simulink model "quadplane_control_dev"  (R2023a)
settings: Solver=FixedStepAuto  StartTime=0.0  StopTime=10.0  FixedStep=0.01  RelTol=1e-3
undefined symbols (not defined in the file or in its folder): Aircraft, DiscIntNeverNeededParam, framePeriod_s, frameRate_hz, InitCond
libraries: simulink x8, eeGeneralControl x6, slpidlib x3, fuzblock x1
(part 2 of 3)

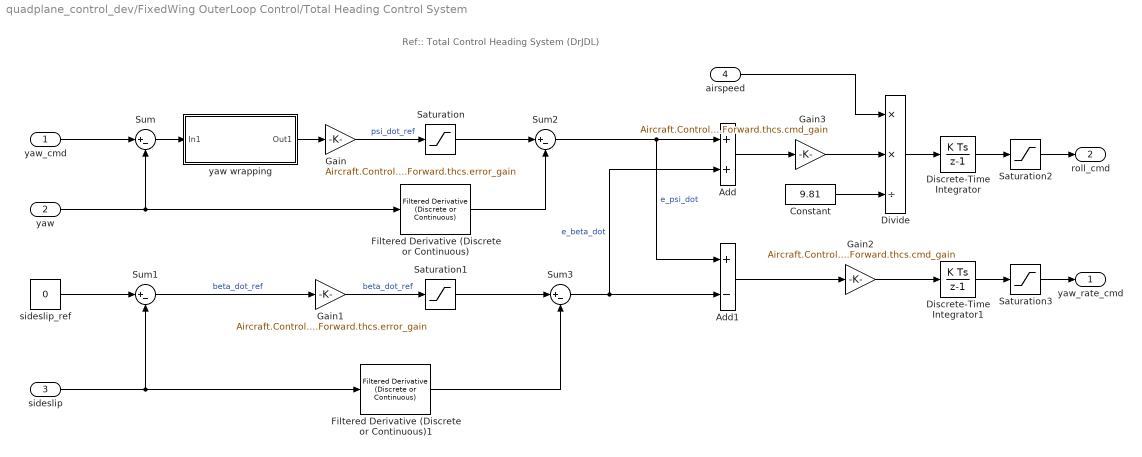
== system quadplane_control_dev/FixedWing OuterLoop Control/Total Heading Control System ==
  note: Ref:: Total Control Heading System (DrJDL)
  yaw_cmd : Inport
  yaw : Inport  Port=2
  sideslip : Inport  Port=3
  airspeed : Inport  Port=4
  " yaw wrapping" : Subsystem
  Add : Sum
  Add1 : Sum  Inputs=+-
  Constant : Constant  Value=9.81  OutDataTypeStr=single
  Discrete-Time Integrator : DiscreteIntegrator  SampleTime=-1  ICPrevOutput=DiscIntNeverNeededParam  ICPrevScaledInput=DiscIntNeverNeededParam
  Discrete-Time Integrator1 : DiscreteIntegrator  SampleTime=-1  ICPrevOutput=DiscIntNeverNeededParam  ICPrevScaledInput=DiscIntNeverNeededParam
  Divide : Product  Inputs=**/
  Filtered Derivative (Discrete or Continuous) : eeGeneralControl/Filtered Derivative (Discrete or Continuous)  K=1  T=0.1  B=inf  A=-inf  minRatio=10  init_option=Inherited from block input  x0=0  Ts=-1
      settings: LibrarySourceBlock=|
      | ee_sl_lib/General Control/Filtered Derivative
      | (Discrete or Continuous)
  Filtered Derivative (Discrete or Continuous)1 : eeGeneralControl/Filtered Derivative (Discrete or Continuous)  K=1  T=0.05  B=inf  A=-inf  minRatio=10  init_option=Inherited from block input  x0=0  Ts=-1
      settings: LibrarySourceBlock=|
      | ee_sl_lib/General Control/Filtered Derivative
      | (Discrete or Continuous)
  Gain : Gain  Gain=Aircraft.Control.Forward.thcs.error_gain
  Gain1 : Gain  Gain=Aircraft.Control.Forward.thcs.error_gain
  Gain2 : Gain  Gain=Aircraft.Control.Forward.thcs.cmd_gain
  Gain3 : Gain  Gain=Aircraft.Control.Forward.thcs.cmd_gain
  Saturation : Saturate  UpperLimit=Aircraft.Control.Forward.thcs.psi_dot_ref  LowerLimit=-Aircraft.Control.Forward.thcs.psi_dot_ref  OutDataTypeStr=single
  Saturation1 : Saturate  UpperLimit=Aircraft.Control.Forward.thcs.beta_dot_ref_limit  LowerLimit=-Aircraft.Control.Forward.thcs.beta_dot_ref_limit  OutDataTypeStr=single
  Saturation2 : Saturate  UpperLimit=Aircraft.Control.Forward.max_roll_rad  LowerLimit=-Aircraft.Control.Forward.max_roll_rad  OutDataTypeStr=single
  Saturation3 : Saturate  UpperLimit=Aircraft.Control.Forward.max_yaw_rate  LowerLimit=-Aircraft.Control.Forward.max_yaw_rate  OutDataTypeStr=single
  Sum{,1..3} (4 alike) : Sum  Inputs=|+-
  sideslip_ref : Constant  Value=0  OutDataTypeStr=single
  yaw_rate_cmd : Outport
  roll_cmd : Outport  Port=2
  wires:
  yaw_cmd/1 -> Sum/1
  yaw/1 -> Filtered Derivative (Discrete or Continuous)/1, Sum/2
  Sum/1 -> " yaw wrapping"/1(In1)
  sideslip_ref/1 -> Sum1/1
  sideslip/1 -> Filtered Derivative (Discrete or Continuous)1/1, Sum1/2
  Gain/1 -> Saturation/1  "psi_dot_ref"
  Gain1/1 -> Saturation1/1  "beta_dot_ref"
  Saturation/1 -> Sum2/1
  Filtered Derivative (Discrete or Continuous)/1 -> Sum2/2
  Sum2/1 -> Add1/1, Add/1  "e_psi_dot"
  Saturation1/1 -> Sum3/1
  Filtered Derivative (Discrete or Continuous)1/1 -> Sum3/2
  Sum3/1 -> Add/2, Add1/2  "e_beta_dot"
  Add1/1 -> Gain2/1
  Gain2/1 -> Discrete-Time Integrator1/1
  Discrete-Time Integrator1/1 -> Saturation3/1
  Add/1 -> Gain3/1
  Gain3/1 -> Divide/2
  Constant/1 -> Divide/3
  Divide/1 -> Discrete-Time Integrator/1
  airspeed/1 -> Divide/1
  Discrete-Time Integrator/1 -> Saturation2/1
  " yaw wrapping"/1(Out1) -> Gain/1
  Saturation2/1 -> roll_cmd/1
  Saturation3/1 -> yaw_rate_cmd/1
  Sum1/1 -> Gain1/1  "beta_dot_ref"

== system quadplane_control_dev/Hover Inner Loop/Attitude Control ==
  note: Limiting the pqr_ref to 2/-2 radps
  yaw_rate_ref : Inport
  roll_pitch_ref : Inport  Port=2
  roll_pitch_yaw : Inport  Port=3
  Gain1 : Gain  Gain=Aircraft.Control.Hover_v2.att_gain
  Mux : Mux  Inputs=2
  Saturation : Saturate  UpperLimit=Aircraft.Control.Hover.pqr_limit  LowerLimit=-Aircraft.Control.Hover.pqr_limit
  Selector : Selector  InputPortWidth=3  IndexOptions=Index vector (dialog)  Indices=[1 2]  OutputSizes=1
  Sum : Sum  Inputs=|+-  AccumDataTypeStr=single
  pqr_ref1 : Outport
  wires:
  roll_pitch_ref/1 -> Sum/1
  Sum/1 -> Gain1/1  "roll_pitch_err"
  Mux/1 -> Saturation/1
  Saturation/1 -> pqr_ref1/1
  Selector/1 -> Sum/2
  roll_pitch_yaw/1 -> Selector/1
  Gain1/1 -> Mux/1
  yaw_rate_ref/1 -> Mux/2

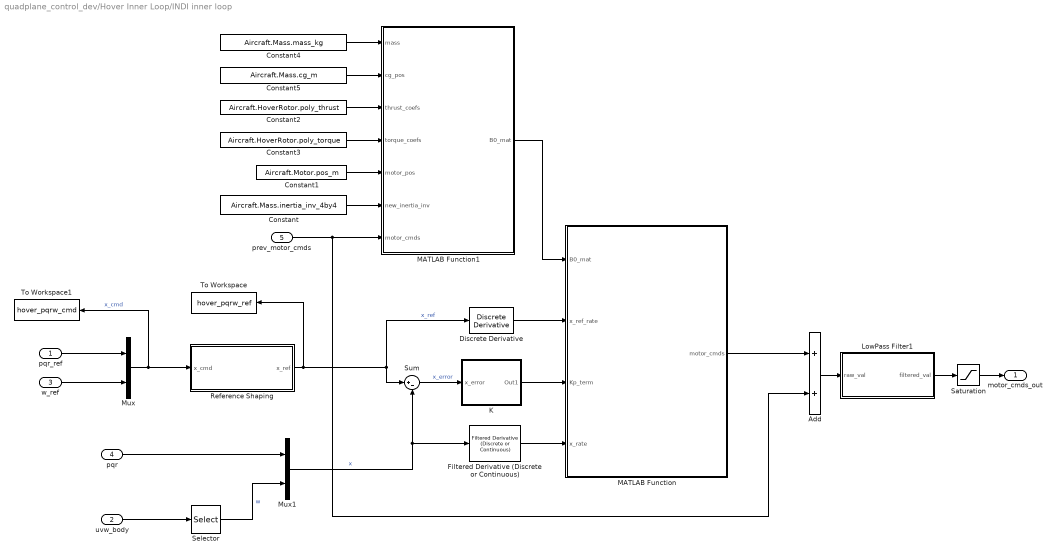
== system quadplane_control_dev/Hover Inner Loop/INDI inner loop ==
  pqr_ref : Inport
  uvw_body : Inport  Port=2
  w_ref : Inport  Port=3
  pqr : Inport  Port=4
  prev_motor_cmds : Inport  Port=5
  Add : Sum
  Constant : Constant  Value=Aircraft.Mass.inertia_inv_4by4  OutDataTypeStr=single
  Constant1 : Constant  Value=Aircraft.Motor.pos_m  OutDataTypeStr=single
  Constant2 : Constant  Value=Aircraft.HoverRotor.poly_thrust  OutDataTypeStr=single
  Constant3 : Constant  Value=Aircraft.HoverRotor.poly_torque  OutDataTypeStr=single
  Constant4 : Constant  Value=Aircraft.Mass.mass_kg
  Constant5 : Constant  Value=Aircraft.Mass.cg_m
  Discrete Derivative : simulink/Discrete/Discrete Derivative  gainval=1.0  ICPrevScaledInput=0.0  OutMin=[]  OutMax=[]  OutDataType=fixdt(1, 16)  OutScaling=2^-10  DoSatur=off
  Filtered Derivative (Discrete or Continuous) : eeGeneralControl/Filtered Derivative (Discrete or Continuous)  K=1  T=0.01  B=inf  A=-inf  minRatio=10  init_option=Inherited from block input  x0=0  Ts=-1
      settings: LibrarySourceBlock=|
      | ee_sl_lib/General Control/Filtered Derivative
      | (Discrete or Continuous)
  K : Subsystem
  LowPass Filter1 : Subsystem
      settings: PortSchema="{\"entries\":[{\"content\":{\"sides\":[{\"content\":{\"connectorIds\":[\"Out1\"]},\"type\":\"ConnectorPlacement.EquallySpacedRectSide\",\"uuid\":\"91cc3e13-2b14-472d-8884-d1975898cd34\"},{\"content\":{\"connectorIds\":[\"In1\"],\"side\":\"RIGHT\"},\"type\":\"ConnectorPlacement.EquallySpacedRectSide\",\"uuid\":\"ce6b3021-6e32-4737-8c8e-25014706d3dd\"},{\"content\":{\"side\":\"TOP\"},\"type\":\"ConnectorPlacement.EquallySpacedRectSide\",\"uuid\":\"ad734f0b-b067-43e6-a641-0e0955250a7f\"},{\"content\":{\"side\":\"BOTTOM\"},\"type\":\"ConnectorPlacement.EquallySpacedRectSide\",\"uuid\":\"618c62c8-d4e2-4678-9fe1-905e2f147d5d\"}]},\"type\":\"ConnectorPlacement.EquallySpacedConnector\",\"uuid\":\"c0097053-d36a-473a-84fb-0616f69f4bc5\"}],\"packageUris\":[\"http://schema.mathworks.com/mf0/Connector/R2020b\"],\"version\":\"1.0\"}"
  MATLAB Function : MATLAB Function  TreatAsAtomicUnit=on
  MATLAB Function1 : MATLAB Function  TreatAsAtomicUnit=on
  Mux : Mux  Inputs=2
  Mux1 : Mux  Inputs=2
  Reference Shaping : Subsystem
  Saturation : Saturate  UpperLimit=1  LowerLimit=0.2
  Selector : Selector  InputPortWidth=3  IndexOptions=Index vector (dialog)  Indices=3  OutputSizes=1
  Sum : Sum  Inputs=|+-  OutDataTypeStr=single
  To Workspace : ToWorkspace  VariableName=hover_pqrw_ref  SaveFormat=Timeseries  SampleTime=-1
  To Workspace1 : ToWorkspace  VariableName=hover_pqrw_cmd  SaveFormat=Timeseries  SampleTime=-1
  motor_cmds_out : Outport
  wires:
  Constant2/1 -> MATLAB Function1/3(thrust_coefs)
  MATLAB Function/1(motor_cmds) -> Add/1
  uvw_body/1 -> Selector/1
  Discrete Derivative/1 -> MATLAB Function/2(x_ref_rate)
  Constant4/1 -> MATLAB Function1/1(mass)
  Constant3/1 -> MATLAB Function1/4(torque_coefs)
  pqr_ref/1 -> Mux/1
  pqr/1 -> Mux1/1
  Constant1/1 -> MATLAB Function1/5(motor_pos)
  Mux1/1 -> Filtered Derivative (Discrete or Continuous)/1, Sum/2  "x"
  Constant/1 -> MATLAB Function1/6(new_inertia_inv)
  MATLAB Function1/1(B0_mat) -> MATLAB Function/1(B0_mat)
  Constant5/1 -> MATLAB Function1/2(cg_pos)
  Selector/1 -> Mux1/2  "w"
  w_ref/1 -> Mux/2
  Reference Shaping/1(x_ref) -> To Workspace/1, Discrete Derivative/1, Sum/1  "x_ref"
  Filtered Derivative (Discrete or Continuous)/1 -> MATLAB Function/4(x_rate)
  Mux/1 -> To Workspace1/1, Reference Shaping/1(x_cmd)  "x_cmd"
  Saturation/1 -> motor_cmds_out/1
  Add/1 -> LowPass Filter1/1(raw_val)
  prev_motor_cmds/1 -> Add/2, MATLAB Function1/7(motor_cmds)
  Sum/1 -> K/1(x_error)  "x_error"
  K/1(Out1) -> MATLAB Function/3(Kp_term)
  LowPass Filter1/1(filtered_val) -> Saturation/1

== system quadplane_control_dev/Hover Outer Loop/Altitude Control ==
  rpy : Inport
  alt_cmd : Inport  Port=2
  alt : Inport  Port=3
  Gain : Gain  Gain=-1
  Gain1 : Gain  Gain=Aircraft.Control.Hover_v2.alt_gain
  MATLAB Function : MATLAB Function  TreatAsAtomicUnit=on
  Saturation : Saturate  UpperLimit=Aircraft.Control.Hover.body_vert_limits(1)  LowerLimit=Aircraft.Control.Hover.body_vert_limits(2)
  Saturation1 : Saturate  UpperLimit=Aircraft.Control.Hover.nav_vert_limits(1)  LowerLimit=Aircraft.Control.Hover.nav_vert_limits(2)
  Sum : Sum  Inputs=|+-
  w_cmd : Outport
  wires:
  Gain/1 -> Saturation1/1
  alt/1 -> Sum/2
  alt_cmd/1 -> Sum/1
  Sum/1 -> Gain1/1
  Gain1/1 -> Gain/1
  rpy/1 -> MATLAB Function/1(roll_pitch)
  Saturation/1 -> w_cmd/1
  MATLAB Function/1(w_ref) -> Saturation/1
  Saturation1/1 -> MATLAB Function/2(z_dot_nav_ref)

== system quadplane_control_dev/Hover Outer Loop/Conditioning ==
  mode : Inport
  roll_pitch_ref : Inport  Port=2
  airspeed_cmd : Inport  Port=3
  speed_up_bool : Inport  Port=4
  Constant : Constant  Value=0  OutDataTypeStr=single
  Constant1 : Constant  Value=[6, 12]  OutDataTypeStr=single
  Demux : Demux  Outputs=2
  MATLAB Function : MATLAB Function  TreatAsAtomicUnit=on
  Mux : Mux  Inputs=2
  Switch : Switch  Criteria=u2 > Threshold  SaturateOnIntegerOverflow=off  InputSameDT=off
  y : Outport
  wires:
  Constant/1 -> Switch/1
  roll_pitch_ref/1 -> Demux/1
  Switch/1 -> Mux/1
  Demux/2 -> Mux/2
  Demux/1 -> Switch/3
  Mux/1 -> MATLAB Function/1(u)
  mode/1 -> Switch/2
  speed_up_bool/1 -> MATLAB Function/3(speed_up_bool)
  MATLAB Function/1(y) -> y/1
  Constant1/1 -> MATLAB Function/4(airspeed_cutoffs)
  airspeed_cmd/1 -> MATLAB Function/2(airspeed_cmd)

== system quadplane_control_dev/Hover Outer Loop/Linear Heading Controller ==
  note: P-gain for Heading Control
  Ground_track_cmd : Inport
  rpy : Inport  Port=2
  Gain : Gain  Gain=Aircraft.Control.Hover_v2.heading_gain
  Loop Protection : Subsystem
  Saturation : Saturate  UpperLimit=Aircraft.Control.Hover_v2.yaw_rate_ref_limit  LowerLimit=-Aircraft.Control.Hover_v2.yaw_rate_ref_limit  OutDataTypeStr=single
  Selector2 : Selector  InputPortWidth=3  IndexOptions=Index vector (dialog)  Indices=3  OutputSizes=1
  Sum : Sum  Inputs=|+-
  yaw_ref_rate : Outport
  wires:
  Ground_track_cmd/1 -> Sum/1
  rpy/1 -> Selector2/1
  Selector2/1 -> Sum/2
  Gain/1 -> Saturation/1
  Saturation/1 -> yaw_ref_rate/1
  Sum/1 -> Loop Protection/1(In1)
  Loop Protection/1(Out1) -> Gain/1

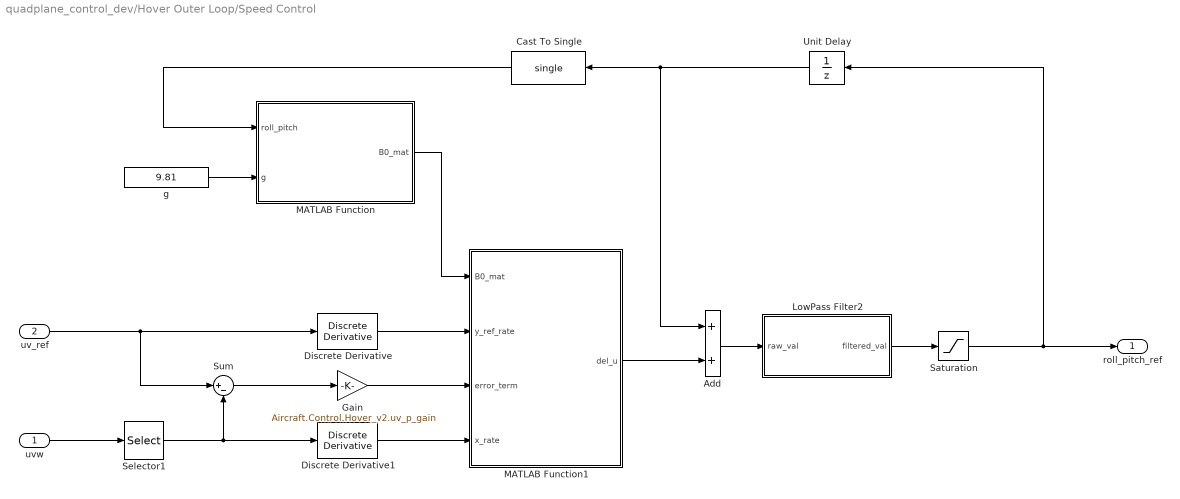
== system quadplane_control_dev/Hover Outer Loop/Speed Control ==
  uvw : Inport
  uv_ref : Inport  Port=2
  Add : Sum
  Cast To Single : DataTypeConversion  OutDataTypeStr=single  SaturateOnIntegerOverflow=off  RndMeth=Floor
  Discrete Derivative : simulink/Discrete/Discrete Derivative  gainval=1.0  ICPrevScaledInput=0.0  OutMin=[]  OutMax=[]  OutDataType=fixdt(1, 16)  OutScaling=2^-10  DoSatur=off
  Discrete Derivative1 : simulink/Discrete/Discrete Derivative  gainval=1.0  ICPrevScaledInput=0.0  OutMin=[]  OutMax=[]  OutDataType=fixdt(1, 16)  OutScaling=2^-10  DoSatur=off
  Gain : Gain  Gain=Aircraft.Control.Hover_v2.uv_p_gain
  LowPass Filter2 : Subsystem
      settings: PortSchema="{\"entries\":[{\"content\":{\"sides\":[{\"content\":{\"connectorIds\":[\"Out1\"]},\"type\":\"ConnectorPlacement.EquallySpacedRectSide\",\"uuid\":\"91cc3e13-2b14-472d-8884-d1975898cd34\"},{\"content\":{\"connectorIds\":[\"In1\"],\"side\":\"RIGHT\"},\"type\":\"ConnectorPlacement.EquallySpacedRectSide\",\"uuid\":\"ce6b3021-6e32-4737-8c8e-25014706d3dd\"},{\"content\":{\"side\":\"TOP\"},\"type\":\"ConnectorPlacement.EquallySpacedRectSide\",\"uuid\":\"ad734f0b-b067-43e6-a641-0e0955250a7f\"},{\"content\":{\"side\":\"BOTTOM\"},\"type\":\"ConnectorPlacement.EquallySpacedRectSide\",\"uuid\":\"618c62c8-d4e2-4678-9fe1-905e2f147d5d\"}]},\"type\":\"ConnectorPlacement.EquallySpacedConnector\",\"uuid\":\"c0097053-d36a-473a-84fb-0616f69f4bc5\"}],\"packageUris\":[\"http://schema.mathworks.com/mf0/Connector/R2020b\"],\"version\":\"1.0\"}"
  MATLAB Function : MATLAB Function  TreatAsAtomicUnit=on
  MATLAB Function1 : MATLAB Function  TreatAsAtomicUnit=on
  Saturation : Saturate  UpperLimit=Aircraft.Control.Hover.roll_pitch_ref_limits'  LowerLimit=-Aircraft.Control.Hover.roll_pitch_ref_limits'
  Selector1 : Selector  InputPortWidth=3  IndexOptions=Index vector (dialog)  Indices=[1 2]  OutputSizes=1
  Sum : Sum  Inputs=|+-
  Unit Delay : UnitDelay  SampleTime=-1  HasFrameUpgradeWarning=on
  g : Constant  Value=9.81  OutDataTypeStr=single
  roll_pitch_ref : Outport
  wires:
  Saturation/1 -> Unit Delay/1, roll_pitch_ref/1
  g/1 -> MATLAB Function/2(g)
  uvw/1 -> Selector1/1
  Selector1/1 -> Discrete Derivative1/1, Sum/2
  Sum/1 -> Gain/1
  Gain/1 -> MATLAB Function1/3(error_term)
  MATLAB Function/1(B0_mat) -> MATLAB Function1/1(B0_mat)
  MATLAB Function1/1(del_u) -> Add/2
  Unit Delay/1 -> Add/1, Cast To Single/1
  Add/1 -> LowPass Filter2/1(raw_val)
  Discrete Derivative1/1 -> MATLAB Function1/4(x_rate)
  Cast To Single/1 -> MATLAB Function/1(roll_pitch)
  Discrete Derivative/1 -> MATLAB Function1/2(y_ref_rate)
  LowPass Filter2/1(filtered_val) -> Saturation/1
  uv_ref/1 -> Sum/1, Discrete Derivative/1

== system quadplane_control_dev/LowPass Filter2/LP Filter on throttle outputs ==
  raw_val : Inport
  freq_cut : Inport  Port=2
  Constant : Constant  Value=frameRate_hz  OutDataTypeStr=single
  MATLAB Function : MATLAB Function  TreatAsAtomicUnit=on
  Unit Delay : UnitDelay  SampleTime=-1  HasFrameUpgradeWarning=on
  filtered_val : Outport
  wires:
  freq_cut/1 -> MATLAB Function/3(freq_cut)
  MATLAB Function/1(filtered_val) -> Unit Delay/1, filtered_val/1
  Unit Delay/1 -> MATLAB Function/1(prev_val)
  raw_val/1 -> MATLAB Function/2(raw_val)
  Constant/1 -> MATLAB Function/4(samp_freq)

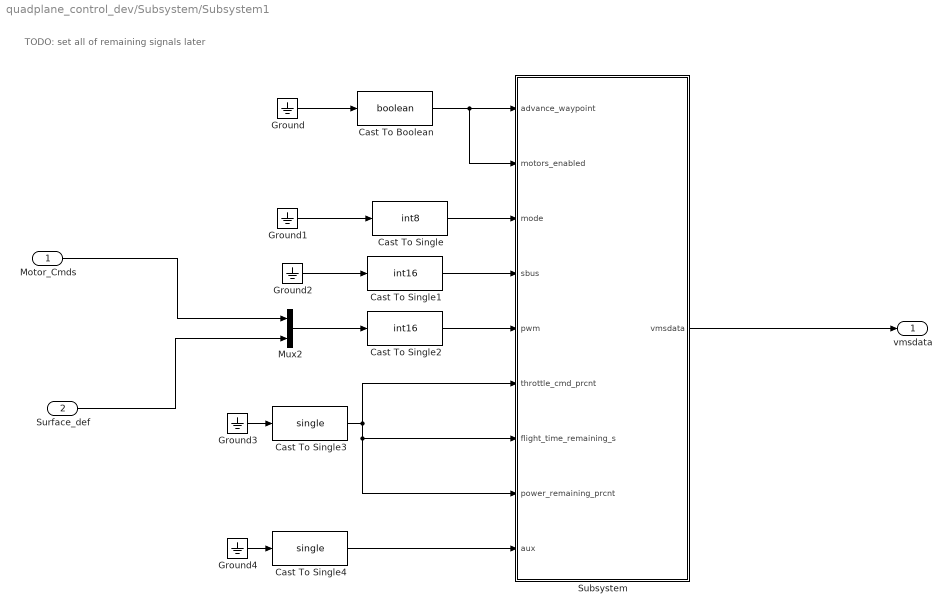
== system quadplane_control_dev/Subsystem/Subsystem1 ==
  note: TODO: set all of remaining signals later
  Motor_Cmds : Inport
  Surface_def : Inport  Port=2
  Cast To Boolean : DataTypeConversion  OutDataTypeStr=boolean  SaturateOnIntegerOverflow=off  RndMeth=Floor
  Cast To Single : DataTypeConversion  OutDataTypeStr=int8  SaturateOnIntegerOverflow=off  RndMeth=Floor
  Cast To Single1 : DataTypeConversion  OutDataTypeStr=int16  SaturateOnIntegerOverflow=off  RndMeth=Floor
  Cast To Single2 : DataTypeConversion  OutDataTypeStr=int16  SaturateOnIntegerOverflow=off  RndMeth=Floor
  Cast To Single3 : DataTypeConversion  OutDataTypeStr=single  SaturateOnIntegerOverflow=off  RndMeth=Floor
  Cast To Single4 : DataTypeConversion  OutDataTypeStr=single  SaturateOnIntegerOverflow=off  RndMeth=Floor
  Ground{,1..4} (5 alike) : Ground
  Mux2 : Mux  Inputs=2
  Subsystem : Subsystem
  vmsdata : Outport
  wires:
  Cast To Single/1 -> Subsystem/3(mode)
  Ground3/1 -> Cast To Single3/1
  Motor_Cmds/1 -> Mux2/1
  Cast To Single3/1 -> Subsystem/6(throttle_cmd_prcnt), Subsystem/8(power_remaining_prcnt), Subsystem/7(flight_time_remaining_s)
  Ground2/1 -> Cast To Single1/1
  Ground1/1 -> Cast To Single/1
  Cast To Single2/1 -> Subsystem/5(pwm)
  Cast To Single1/1 -> Subsystem/4(sbus)
  Surface_def/1 -> Mux2/2
  Cast To Single4/1 -> Subsystem/9(aux)
  Ground4/1 -> Cast To Single4/1
  Subsystem/1(vmsdata) -> vmsdata/1
  Ground/1 -> Cast To Boolean/1
  Cast To Boolean/1 -> Subsystem/2(motors_enabled), Subsystem/1(advance_waypoint)
  Mux2/1 -> Cast To Single2/1

== system quadplane_control_dev/Subsystem/deflections_PWM_denormalize ==
  note: Remap to PWM signal
  normalized_input : Inport
  Constant : Constant  Value=Aircraft.Surf.Limit.neg_deg(1)  OutDataTypeStr=single
  Constant1 : Constant  Value=1100  OutDataTypeStr=single
  Constant2 : Constant  Value=1950  OutDataTypeStr=single
  Constant3 : Constant  Value=Aircraft.Surf.Limit.pos_deg(1)  OutDataTypeStr=single
  remap : MATLAB Function  TreatAsAtomicUnit=on
  raw_output : Outport
  wires:
  Constant2/1 -> remap/5(out_max)
  Constant1/1 -> remap/4(out_min)
  Constant3/1 -> remap/3(in_max)
  Constant/1 -> remap/2(in_min)
  remap/1(raw_out) -> raw_output/1
  normalized_input/1 -> remap/1(norm_in)

== system quadplane_control_dev/Subsystem/motor_PWM_denormalize ==
  note: Remap to PWM signal
  normalized_input : Inport
  Constant : Constant  Value=0  OutDataTypeStr=single
  Constant1 : Constant  Value=1100  OutDataTypeStr=single
  Constant2 : Constant  Value=1950  OutDataTypeStr=single
  Constant3 : Constant  OutDataTypeStr=single
  remap : MATLAB Function  TreatAsAtomicUnit=on
  raw_output : Outport
  wires:
  Constant2/1 -> remap/5(out_max)
  Constant1/1 -> remap/4(out_min)
  Constant3/1 -> remap/3(in_max)
  Constant/1 -> remap/2(in_min)
  remap/1(raw_out) -> raw_output/1
  normalized_input/1 -> remap/1(norm_in)

== system quadplane_control_dev/Subsystem1/LowPass Filter1 ==
  raw_val : Inport
  Constant : Constant  Value=Aircraft.Control.Hover.u_ref_LP_filter_CTOFF
  LP Filter on throttle outputs : Subsystem
      settings: PortSchema="{\"entries\":[{\"content\":{\"sides\":[{\"content\":{\"connectorIds\":[\"In1\"]},\"type\":\"ConnectorPlacement.EquallySpacedRectSide\",\"uuid\":\"20236834-aeb3-4c5b-bb2e-f84447e752b5\"},{\"content\":{\"connectorIds\":[\"Out1\"],\"side\":\"RIGHT\"},\"type\":\"ConnectorPlacement.EquallySpacedRectSide\",\"uuid\":\"d668f9a1-a3df-4207-8bf1-99fb838e59b2\"},{\"content\":{\"connectorIds\":[],\"side\":\"TOP\"},\"type\":\"ConnectorPlacement.EquallySpacedRectSide\",\"uuid\":\"66cceb06-f4bc-4278-b965-2427292e46df\"},{\"content\":{\"connectorIds\":[\"In2\"],\"side\":\"BOTTOM\"},\"type\":\"ConnectorPlacement.EquallySpacedRectSide\",\"uuid\":\"8fdaac6a-cb03-4bd4-87bb-7bafd10bc297\"}]},\"type\":\"ConnectorPlacement.EquallySpacedConnector\",\"uuid\":\"3dc29a9a-e794-478d-b7df-452e6c2d3f66\"}],\"packageUris\":[\"http://schema.mathworks.com/mf0/Connector/R2020b\"],\"version\":\"1.0\"}"
  filtered_val : Outport
  wires:
  raw_val/1 -> LP Filter on throttle outputs/1(raw_val)
  Constant/1 -> LP Filter on throttle outputs/2(freq_cut)
  LP Filter on throttle outputs/1(filtered_val) -> filtered_val/1

== system quadplane_control_dev/Subsystem5/LowPass Filter1 ==
  raw_val : Inport
  Constant : Constant  Value=0.1
  LP Filter on throttle outputs : Subsystem
      settings: PortSchema="{\"entries\":[{\"content\":{\"sides\":[{\"content\":{\"connectorIds\":[\"In1\"]},\"type\":\"ConnectorPlacement.EquallySpacedRectSide\",\"uuid\":\"20236834-aeb3-4c5b-bb2e-f84447e752b5\"},{\"content\":{\"connectorIds\":[\"Out1\"],\"side\":\"RIGHT\"},\"type\":\"ConnectorPlacement.EquallySpacedRectSide\",\"uuid\":\"d668f9a1-a3df-4207-8bf1-99fb838e59b2\"},{\"content\":{\"connectorIds\":[],\"side\":\"TOP\"},\"type\":\"ConnectorPlacement.EquallySpacedRectSide\",\"uuid\":\"66cceb06-f4bc-4278-b965-2427292e46df\"},{\"content\":{\"connectorIds\":[\"In2\"],\"side\":\"BOTTOM\"},\"type\":\"ConnectorPlacement.EquallySpacedRectSide\",\"uuid\":\"8fdaac6a-cb03-4bd4-87bb-7bafd10bc297\"}]},\"type\":\"ConnectorPlacement.EquallySpacedConnector\",\"uuid\":\"3dc29a9a-e794-478d-b7df-452e6c2d3f66\"}],\"packageUris\":[\"http://schema.mathworks.com/mf0/Connector/R2020b\"],\"version\":\"1.0\"}"
  filtered_val : Outport
  wires:
  raw_val/1 -> LP Filter on throttle outputs/1(raw_val)
  Constant/1 -> LP Filter on throttle outputs/2(freq_cut)
  LP Filter on throttle outputs/1(filtered_val) -> filtered_val/1

== system quadplane_control_dev/Trajectory Command/Subsystem ==
  Mux : Mux  Inputs=2
  Step4 : Step  Time=73  After=3  OutDataTypeStr=single  SampleTime=0
  Step5 : Step  Time=27  After=0  OutDataTypeStr=single  SampleTime=0
  uv_ref_hover : Outport
  wires:
  Step5/1 -> Mux/1
  Mux/1 -> uv_ref_hover/1
  Step4/1 -> Mux/2

== system quadplane_control_dev/Trajectory Command/Subsystem1 ==
  Add3 : Sum  Inputs=++++
  Constant3 : Constant  Value=0.3  OutDataTypeStr=single
  Step3 : Step  Time=2  After=-0.8  OutDataTypeStr=single  SampleTime=0
  Step7 : Step  Time=18  Before=-0.8  After=0.5  OutDataTypeStr=single  SampleTime=0
  Step8 : Step  Time=30  Before=0.5  After=2.75  OutDataTypeStr=single  SampleTime=0
  hdg_cmd : Outport
  wires:
  Step7/1 -> Add3/2
  Step8/1 -> Add3/4
  Constant3/1 -> Add3/3
  Add3/1 -> hdg_cmd/1
  Step3/1 -> Add3/1

== system quadplane_control_dev/Trajectory Command/Subsystem2 ==
  mode_input : Inport
  Constant : Constant  Value=0  OutDataTypeStr=single
  Ramp1 : simulink/Sources/Ramp  slope=Aircraft.Control.modes.hover2forward_airspeed_ramp  start=7  InitialOutput=0
  Ramp2 : simulink/Sources/Ramp  slope=Aircraft.Control.modes.forward2hover_airspeed_ramp  start=52  InitialOutput=0
  Saturation1 : Saturate  UpperLimit=22  LowerLimit=0  OutDataTypeStr=single
  Saturation2 : Saturate  UpperLimit=22  LowerLimit=0  OutDataTypeStr=single
  Scope4 : Scope
  Sum : Sum  Inputs=|++
  Switch : Switch  Criteria=u2 > Threshold  SaturateOnIntegerOverflow=off  InputSameDT=off
  airspeed_cmd : Outport
  wires:
  Ramp1/1 -> Saturation1/1
  Constant/1 -> Switch/3
  Ramp2/1 -> Sum/2
  Saturation2/1 -> Switch/1, Scope4/1
  Sum/1 -> Saturation2/1
  Saturation1/1 -> Sum/1
  mode_input/1 -> Switch/2
  Switch/1 -> airspeed_cmd/1

== system quadplane_control_dev/Trajectory Command/Subsystem3 ==
  Step2 : Step  Time=48  Before=100  After=90  OutDataTypeStr=single  SampleTime=0
  altitude_cmd : Outport
  wires:
  Step2/1 -> altitude_cmd/1

== system quadplane_control_dev/Trajectory Command/Subsystem4 ==
  Add1 : Sum  Inputs=+++++
  Constant1 : Constant  Value=-4
  Step : Step  Time=7  SampleTime=0
  Step1 : Step  Time=18  Before=1  After=2  SampleTime=0
  Step2 : Step  Time=52  Before=2  SampleTime=0
  Step3 : Step  Time=70  Before=1  After=0  SampleTime=0
  mode_input : Outport
  wires:
  Step2/1 -> Add1/2
  Constant1/1 -> Add1/5
  Step1/1 -> Add1/4
  Step3/1 -> Add1/3
  Step/1 -> Add1/1
  Add1/1 -> mode_input/1

== system quadplane_control_dev/Check if speeding up/LowPass Filter/LP Filter on Accel ==
  raw_val : Inport
  freq_cut : Inport  Port=2
  Constant : Constant  Value=frameRate_hz  OutDataTypeStr=single
  MATLAB Function : MATLAB Function  TreatAsAtomicUnit=on
  Unit Delay : UnitDelay  SampleTime=-1  HasFrameUpgradeWarning=on
  filtered_val : Outport
  wires:
  freq_cut/1 -> MATLAB Function/3(freq_cut)
  MATLAB Function/1(filtered_val) -> Unit Delay/1, filtered_val/1
  Unit Delay/1 -> MATLAB Function/1(prev_val)
  raw_val/1 -> MATLAB Function/2(raw_val)
  Constant/1 -> MATLAB Function/4(samp_freq)

== system quadplane_control_dev/FixedWing InnerLoop Control/INDI Based Angular Rate Controller/LowPass Filter1 ==
  raw_val : Inport
  Constant : Constant
  LP Filter on throttle outputs : Subsystem
      settings: PortSchema="{\"entries\":[{\"content\":{\"sides\":[{\"content\":{\"connectorIds\":[\"In1\"]},\"type\":\"ConnectorPlacement.EquallySpacedRectSide\",\"uuid\":\"20236834-aeb3-4c5b-bb2e-f84447e752b5\"},{\"content\":{\"connectorIds\":[\"Out1\"],\"side\":\"RIGHT\"},\"type\":\"ConnectorPlacement.EquallySpacedRectSide\",\"uuid\":\"d668f9a1-a3df-4207-8bf1-99fb838e59b2\"},{\"content\":{\"connectorIds\":[],\"side\":\"TOP\"},\"type\":\"ConnectorPlacement.EquallySpacedRectSide\",\"uuid\":\"66cceb06-f4bc-4278-b965-2427292e46df\"},{\"content\":{\"connectorIds\":[\"In2\"],\"side\":\"BOTTOM\"},\"type\":\"ConnectorPlacement.EquallySpacedRectSide\",\"uuid\":\"8fdaac6a-cb03-4bd4-87bb-7bafd10bc297\"}]},\"type\":\"ConnectorPlacement.EquallySpacedConnector\",\"uuid\":\"3dc29a9a-e794-478d-b7df-452e6c2d3f66\"}],\"packageUris\":[\"http://schema.mathworks.com/mf0/Connector/R2020b\"],\"version\":\"1.0\"}"
  filtered_val : Outport
  wires:
  raw_val/1 -> LP Filter on throttle outputs/1(raw_val)
  Constant/1 -> LP Filter on throttle outputs/2(freq_cut)
  LP Filter on throttle outputs/1(filtered_val) -> filtered_val/1

== system quadplane_control_dev/FixedWing InnerLoop Control/INDI Based Angular Rate Controller/Subsystem ==
  pqr_ref : Inport
  Integrator : Integrator
  Integrator1 : Integrator
  K1 : Gain  Gain=Aircraft.Control.Forward_v2.pqr_ref_k1_k2(1)
  K2 : Gain  Gain=Aircraft.Control.Forward_v2.pqr_ref_k1_k2(2)
  Sum : Sum  Inputs=|+-
  Sum1 : Sum  Inputs=|+-
  Out1 : Outport
  wires:
  Sum/1 -> K1/1
  K1/1 -> Sum1/1
  K2/1 -> Integrator/1  "x_dotdot_ref"
  Sum1/1 -> K2/1
  pqr_ref/1 -> Sum/1  "x_cmd"
  Integrator/1 -> Sum1/2, Integrator1/1  "x_dot_ref"
  Integrator1/1 -> Out1/1, Sum/2  "x_ref"

== system quadplane_control_dev/FixedWing OuterLoop Control/INDI Speed & Altitude Controller/LowPass Filter ==
  raw_val : Inport
  Constant : Constant  Value=[1.25, 0.75]  OutDataTypeStr=single
  LP Filter on Accel : Subsystem
      settings: PortSchema="{\"entries\":[{\"content\":{\"sides\":[{\"content\":{\"connectorIds\":[\"In1\"]},\"type\":\"ConnectorPlacement.EquallySpacedRectSide\",\"uuid\":\"20236834-aeb3-4c5b-bb2e-f84447e752b5\"},{\"content\":{\"connectorIds\":[\"Out1\"],\"side\":\"RIGHT\"},\"type\":\"ConnectorPlacement.EquallySpacedRectSide\",\"uuid\":\"d668f9a1-a3df-4207-8bf1-99fb838e59b2\"},{\"content\":{\"connectorIds\":[],\"side\":\"TOP\"},\"type\":\"ConnectorPlacement.EquallySpacedRectSide\",\"uuid\":\"66cceb06-f4bc-4278-b965-2427292e46df\"},{\"content\":{\"connectorIds\":[\"In2\"],\"side\":\"BOTTOM\"},\"type\":\"ConnectorPlacement.EquallySpacedRectSide\",\"uuid\":\"8fdaac6a-cb03-4bd4-87bb-7bafd10bc297\"}]},\"type\":\"ConnectorPlacement.EquallySpacedConnector\",\"uuid\":\"3dc29a9a-e794-478d-b7df-452e6c2d3f66\"}],\"packageUris\":[\"http://schema.mathworks.com/mf0/Connector/R2020b\"],\"version\":\"1.0\"}"
  filtered_val : Outport
  wires:
  raw_val/1 -> LP Filter on Accel/1(raw_val)
  Constant/1 -> LP Filter on Accel/2(freq_cut)
  LP Filter on Accel/1(filtered_val) -> filtered_val/1

== system quadplane_control_dev/FixedWing OuterLoop Control/Total Heading Control System/ yaw wrapping ==
  In1 : Inport
  Abs : Abs  SaturateOnIntegerOverflow=off
  Constant1 : Constant  Value=2*pi  OutDataTypeStr=single
  Product : Product
  Sign : Signum
  Subtract1 : Sum  Inputs=+-
  Switch : Switch  Criteria=u2 > Threshold  Threshold=3.1416  SaturateOnIntegerOverflow=off  InputSameDT=off
  Out1 : Outport
  wires:
  Product/1 -> Subtract1/2
  Switch/1 -> Out1/1
  In1/1 -> Abs/1, Switch/3, Subtract1/1, Sign/1
  Sign/1 -> Product/1
  Constant1/1 -> Product/2
  Subtract1/1 -> Switch/1
  Abs/1 -> Switch/2

== system quadplane_control_dev/Hover Inner Loop/INDI inner loop/K ==
  x_error : Inport
  Add : Sum
  Discrete-Time Integrator : DiscreteIntegrator  SampleTime=-1  ICPrevOutput=DiscIntNeverNeededParam  ICPrevScaledInput=DiscIntNeverNeededParam
  Gain : Gain  Gain=Aircraft.Control.Hover_v2.pq_p_gain  OutDataTypeStr=single
  Gain1 : Gain  Gain=Aircraft.Control.Hover_v2.w_p_gain
  Gain2 : Gain  Gain=Aircraft.Control.Hover_v2.w_i_gain
  Gain3 : Gain  Gain=Aircraft.Control.Hover_v2.r_p_gain
  Mux : Mux  Inputs=3
  Selector : Selector  InputPortWidth=4  IndexOptions=Index vector (dialog)  Indices=[4]  OutputSizes=1
  Selector1 : Selector  InputPortWidth=4  IndexOptions=Index vector (dialog)  Indices=[1 2]  OutputSizes=1
  Selector2 : Selector  InputPortWidth=4  IndexOptions=Index vector (dialog)  Indices=[3]  OutputSizes=1
  Out1 : Outport
  wires:
  Gain/1 -> Mux/1
  x_error/1 -> Selector1/1, Selector/1, Selector2/1
  Selector/1 -> Discrete-Time Integrator/1, Gain1/1  "err_w"
  Selector1/1 -> Gain/1  "err_pq"
  Discrete-Time Integrator/1 -> Gain2/1
  Gain1/1 -> Add/1
  Gain2/1 -> Add/2
  Add/1 -> Mux/3
  Mux/1 -> Out1/1
  Selector2/1 -> Gain3/1  "err_r"
  Gain3/1 -> Mux/2

== system quadplane_control_dev/Hover Inner Loop/INDI inner loop/LowPass Filter1 ==
  raw_val : Inport
  Constant : Constant  Value=0.5
  LP Filter on throttle outputs : Subsystem
      settings: PortSchema="{\"entries\":[{\"content\":{\"sides\":[{\"content\":{\"connectorIds\":[\"In1\"]},\"type\":\"ConnectorPlacement.EquallySpacedRectSide\",\"uuid\":\"20236834-aeb3-4c5b-bb2e-f84447e752b5\"},{\"content\":{\"connectorIds\":[\"Out1\"],\"side\":\"RIGHT\"},\"type\":\"ConnectorPlacement.EquallySpacedRectSide\",\"uuid\":\"d668f9a1-a3df-4207-8bf1-99fb838e59b2\"},{\"content\":{\"connectorIds\":[],\"side\":\"TOP\"},\"type\":\"ConnectorPlacement.EquallySpacedRectSide\",\"uuid\":\"66cceb06-f4bc-4278-b965-2427292e46df\"},{\"content\":{\"connectorIds\":[\"In2\"],\"side\":\"BOTTOM\"},\"type\":\"ConnectorPlacement.EquallySpacedRectSide\",\"uuid\":\"8fdaac6a-cb03-4bd4-87bb-7bafd10bc297\"}]},\"type\":\"ConnectorPlacement.EquallySpacedConnector\",\"uuid\":\"3dc29a9a-e794-478d-b7df-452e6c2d3f66\"}],\"packageUris\":[\"http://schema.mathworks.com/mf0/Connector/R2020b\"],\"version\":\"1.0\"}"
  filtered_val : Outport
  wires:
  raw_val/1 -> LP Filter on throttle outputs/1(raw_val)
  Constant/1 -> LP Filter on throttle outputs/2(freq_cut)
  LP Filter on throttle outputs/1(filtered_val) -> filtered_val/1

== system quadplane_control_dev/Hover Inner Loop/INDI inner loop/Reference Shaping ==
  x_cmd : Inport
  Mux : Mux  Inputs=3
  Selector : Selector  InputPortWidth=4  IndexOptions=Index vector (dialog)  Indices=[1 2]  OutputSizes=1
  Selector1 : Selector  InputPortWidth=4  IndexOptions=Index vector (dialog)  Indices=[3]  OutputSizes=1
  Selector2 : Selector  InputPortWidth=4  IndexOptions=Index vector (dialog)  Indices=[4]  OutputSizes=1
  pqr reference shape : Subsystem
  pqr reference shape1 : Subsystem
  w reference shape : Subsystem
  x_ref : Outport
  wires:
  Selector/1 -> pqr reference shape/1(In1)
  pqr reference shape/1(x_ref) -> Mux/1
  w reference shape/1(x_ref) -> Mux/3
  Mux/1 -> x_ref/1
  x_cmd/1 -> Selector/1, Selector1/1, Selector2/1
  Selector2/1 -> w reference shape/1(In1)
  Selector1/1 -> pqr reference shape1/1(In1)
  pqr reference shape1/1(x_ref) -> Mux/2

== system quadplane_control_dev/Hover Outer Loop/Linear Heading Controller/Loop Protection ==
  In1 : Inport
  Abs : Abs  SaturateOnIntegerOverflow=off
  Constant : Constant  Value=2*pi  OutDataTypeStr=single
  Product : Product
  Sign : Signum
  Subtract1 : Sum  Inputs=+-
  Switch : Switch  Criteria=u2 > Threshold  Threshold=3.1416  SaturateOnIntegerOverflow=off  InputSameDT=off
  Out1 : Outport
  wires:
  Subtract1/1 -> Switch/1
  Constant/1 -> Product/2
  In1/1 -> Abs/1, Switch/3, Subtract1/1, Sign/1
  Product/1 -> Subtract1/2
  Abs/1 -> Switch/2
  Switch/1 -> Out1/1
  Sign/1 -> Product/1

== system quadplane_control_dev/Hover Outer Loop/Speed Control/LowPass Filter2 ==
  raw_val : Inport
  Constant : Constant  Value=Aircraft.Control.Hover_v2.roll_pitch_ref_LP_filter_CTOFF
  LP Filter on throttle outputs : Subsystem
      settings: PortSchema="{\"entries\":[{\"content\":{\"sides\":[{\"content\":{\"connectorIds\":[\"In1\"]},\"type\":\"ConnectorPlacement.EquallySpacedRectSide\",\"uuid\":\"20236834-aeb3-4c5b-bb2e-f84447e752b5\"},{\"content\":{\"connectorIds\":[\"Out1\"],\"side\":\"RIGHT\"},\"type\":\"ConnectorPlacement.EquallySpacedRectSide\",\"uuid\":\"d668f9a1-a3df-4207-8bf1-99fb838e59b2\"},{\"content\":{\"connectorIds\":[],\"side\":\"TOP\"},\"type\":\"ConnectorPlacement.EquallySpacedRectSide\",\"uuid\":\"66cceb06-f4bc-4278-b965-2427292e46df\"},{\"content\":{\"connectorIds\":[\"In2\"],\"side\":\"BOTTOM\"},\"type\":\"ConnectorPlacement.EquallySpacedRectSide\",\"uuid\":\"8fdaac6a-cb03-4bd4-87bb-7bafd10bc297\"}]},\"type\":\"ConnectorPlacement.EquallySpacedConnector\",\"uuid\":\"3dc29a9a-e794-478d-b7df-452e6c2d3f66\"}],\"packageUris\":[\"http://schema.mathworks.com/mf0/Connector/R2020b\"],\"version\":\"1.0\"}"
  filtered_val : Outport
  wires:
  raw_val/1 -> LP Filter on throttle outputs/1(raw_val)
  Constant/1 -> LP Filter on throttle outputs/2(freq_cut)
  LP Filter on throttle outputs/1(filtered_val) -> filtered_val/1

== system quadplane_control_dev/Subsystem/Subsystem1/Subsystem ==
  advance_waypoint : Inport
  motors_enabled : Inport  Port=2
  mode : Inport  Port=3
  sbus : Inport  Port=4
  pwm : Inport  Port=5
  throttle_cmd_prcnt : Inport  Port=6
  flight_time_remaining_s : Inport  Port=7
  power_remaining_prcnt : Inport  Port=8
  aux : Inport  Port=9
  Bus Creator : BusCreator  Inputs=9  OutDataTypeStr=Bus: VmsData  NonVirtualBus=on
      settings: InheritFromInputs=off
  vmsdata : Outport
  wires:
  flight_time_remaining_s/1 -> Bus Creator/7  "flight_time_remaining_s"
  mode/1 -> Bus Creator/3  "mode"
  pwm/1 -> Bus Creator/5  "pwm"
  aux/1 -> Bus Creator/9  "aux"
  throttle_cmd_prcnt/1 -> Bus Creator/6  "throttle_cmd_prcnt"
  Bus Creator/1 -> vmsdata/1
  motors_enabled/1 -> Bus Creator/2  "motors_enabled"
  advance_waypoint/1 -> Bus Creator/1  "advance_waypoint"
  power_remaining_prcnt/1 -> Bus Creator/8  "power_remaining_prcnt"
  sbus/1 -> Bus Creator/4  "sbus"

== system quadplane_control_dev/Subsystem1/LowPass Filter1/LP Filter on throttle outputs ==
  raw_val : Inport
  freq_cut : Inport  Port=2
  Constant : Constant  Value=frameRate_hz  OutDataTypeStr=single
  MATLAB Function : MATLAB Function  TreatAsAtomicUnit=on
  Unit Delay : UnitDelay  SampleTime=-1  HasFrameUpgradeWarning=on
  filtered_val : Outport
  wires:
  freq_cut/1 -> MATLAB Function/3(freq_cut)
  MATLAB Function/1(filtered_val) -> Unit Delay/1, filtered_val/1
  Unit Delay/1 -> MATLAB Function/1(prev_val)
  raw_val/1 -> MATLAB Function/2(raw_val)
  Constant/1 -> MATLAB Function/4(samp_freq)

== system quadplane_control_dev/Subsystem5/LowPass Filter1/LP Filter on throttle outputs ==
  raw_val : Inport
  freq_cut : Inport  Port=2
  Constant : Constant  Value=frameRate_hz  OutDataTypeStr=single
  MATLAB Function : MATLAB Function  TreatAsAtomicUnit=on
  Unit Delay : UnitDelay  SampleTime=-1  HasFrameUpgradeWarning=on
  filtered_val : Outport
  wires:
  freq_cut/1 -> MATLAB Function/3(freq_cut)
  MATLAB Function/1(filtered_val) -> Unit Delay/1, filtered_val/1
  Unit Delay/1 -> MATLAB Function/1(prev_val)
  raw_val/1 -> MATLAB Function/2(raw_val)
  Constant/1 -> MATLAB Function/4(samp_freq)

== system quadplane_control_dev/FixedWing InnerLoop Control/INDI Based Angular Rate Controller/LowPass Filter1/LP Filter on throttle outputs ==
  raw_val : Inport
  freq_cut : Inport  Port=2
  Constant : Constant  Value=frameRate_hz  OutDataTypeStr=single
  MATLAB Function : MATLAB Function  TreatAsAtomicUnit=on
  Unit Delay : UnitDelay  SampleTime=-1  HasFrameUpgradeWarning=on
  filtered_val : Outport
  wires:
  freq_cut/1 -> MATLAB Function/3(freq_cut)
  MATLAB Function/1(filtered_val) -> Unit Delay/1, filtered_val/1
  Unit Delay/1 -> MATLAB Function/1(prev_val)
  raw_val/1 -> MATLAB Function/2(raw_val)
  Constant/1 -> MATLAB Function/4(samp_freq)

== system quadplane_control_dev/FixedWing OuterLoop Control/INDI Speed & Altitude Controller/LowPass Filter/LP Filter on Accel ==
  raw_val : Inport
  freq_cut : Inport  Port=2
  Constant : Constant  Value=frameRate_hz  OutDataTypeStr=single
  MATLAB Function : MATLAB Function  TreatAsAtomicUnit=on
  Unit Delay : UnitDelay  SampleTime=-1  HasFrameUpgradeWarning=on
  filtered_val : Outport
  wires:
  freq_cut/1 -> MATLAB Function/3(freq_cut)
  MATLAB Function/1(filtered_val) -> Unit Delay/1, filtered_val/1
  Unit Delay/1 -> MATLAB Function/1(prev_val)
  raw_val/1 -> MATLAB Function/2(raw_val)
  Constant/1 -> MATLAB Function/4(samp_freq)

== system quadplane_control_dev/Hover Inner Loop/INDI inner loop/LowPass Filter1/LP Filter on throttle outputs ==
  raw_val : Inport
  freq_cut : Inport  Port=2
  Constant : Constant  Value=frameRate_hz  OutDataTypeStr=single
  MATLAB Function : MATLAB Function  TreatAsAtomicUnit=on
  Unit Delay : UnitDelay  SampleTime=-1  HasFrameUpgradeWarning=on
  filtered_val : Outport
  wires:
  freq_cut/1 -> MATLAB Function/3(freq_cut)
  MATLAB Function/1(filtered_val) -> Unit Delay/1, filtered_val/1
  Unit Delay/1 -> MATLAB Function/1(prev_val)
  raw_val/1 -> MATLAB Function/2(raw_val)
  Constant/1 -> MATLAB Function/4(samp_freq)

== system quadplane_control_dev/Hover Inner Loop/INDI inner loop/Reference Shaping/pqr reference shape ==
  In1 : Inport
  Integrator : Integrator
  Integrator1 : Integrator
  K1 : Gain  Gain=Aircraft.Control.Hover_v2.pqr_ref_k1_k2(1)
  K2 : Gain  Gain=Aircraft.Control.Hover_v2.pqr_ref_k1_k2(2)
  Sum1 : Sum  Inputs=|+-
  Sum2 : Sum  Inputs=|+-
  x_ref : Outport
  wires:
  Integrator1/1 -> x_ref/1, Sum1/2  "x_ref"
  Sum2/1 -> K2/1
  Sum1/1 -> K1/1
  Integrator/1 -> Sum2/2, Integrator1/1  "x_dot_ref"
  K1/1 -> Sum2/1
  K2/1 -> Integrator/1  "x_dotdot_ref"
  In1/1 -> Sum1/1

== system quadplane_control_dev/Hover Inner Loop/INDI inner loop/Reference Shaping/pqr reference shape1 ==
  In1 : Inport
  Integrator : Integrator
  Integrator1 : Integrator
  K1 : Gain  Gain=Aircraft.Control.Hover_v2.r_ref_k1_k2(1)
  K2 : Gain  Gain=Aircraft.Control.Hover_v2.r_ref_k1_k2(2)
  Sum1 : Sum  Inputs=|+-
  Sum2 : Sum  Inputs=|+-
  x_ref : Outport
  wires:
  Integrator1/1 -> x_ref/1, Sum1/2  "x_ref"
  Sum2/1 -> K2/1
  Sum1/1 -> K1/1
  Integrator/1 -> Sum2/2, Integrator1/1  "x_dot_ref"
  K1/1 -> Sum2/1
  K2/1 -> Integrator/1  "x_dotdot_ref"
  In1/1 -> Sum1/1

== system quadplane_control_dev/Hover Inner Loop/INDI inner loop/Reference Shaping/w reference shape ==
  In1 : Inport
  Integrator : Integrator
  Integrator1 : Integrator
  K1 : Gain  Gain=Aircraft.Control.Hover_v2.w_ref_k1_k2(1)
  K2 : Gain  Gain=Aircraft.Control.Hover_v2.w_ref_k1_k2(2)
  Sum1 : Sum  Inputs=|+-
  Sum2 : Sum  Inputs=|+-
  x_ref : Outport
  wires:
  Integrator1/1 -> x_ref/1, Sum1/2  "x_ref"
  Sum2/1 -> K2/1
  Sum1/1 -> K1/1
  Integrator/1 -> Sum2/2, Integrator1/1  "x_dot_ref"
  K1/1 -> Sum2/1
  K2/1 -> Integrator/1  "x_dotdot_ref"
  In1/1 -> Sum1/1

== system quadplane_control_dev/Hover Outer Loop/Speed Control/LowPass Filter2/LP Filter on throttle outputs ==
  raw_val : Inport
  freq_cut : Inport  Port=2
  Constant : Constant  Value=frameRate_hz  OutDataTypeStr=single
  MATLAB Function : MATLAB Function  TreatAsAtomicUnit=on
  Unit Delay : UnitDelay  SampleTime=-1  HasFrameUpgradeWarning=on
  filtered_val : Outport
  wires:
  freq_cut/1 -> MATLAB Function/3(freq_cut)
  MATLAB Function/1(filtered_val) -> Unit Delay/1, filtered_val/1
  Unit Delay/1 -> MATLAB Function/1(prev_val)
  raw_val/1 -> MATLAB Function/2(raw_val)
  Constant/1 -> MATLAB Function/4(samp_freq)

== matlab function quadplane_control_dev/FixedWing OuterLoop Control/INDI Speed & Altitude Controller/Compute Inversion Matrix ==
  data: throttle_cmd input; pitch_cmd input single; diam input; B0_mat output single; mass input single; rpm input; density input single; Sref input single; CD_alpha input single; CL_alpha input single; x input single
function B0_mat = inversion_term(throttle_cmd, pitch_cmd, diam, mass, rpm, density, Sref, CD_alpha, CL_alpha, x)

airspeed = x(1);
flight_path = x(2);

% Rough generalizations to make the inversion eqn simpler
RPM = rpm * (2*pi/60);
R = (diam/2) * 0.0254;

% dg/du term from the Taylor series expansion of the state derivative
B0_mat = [(1/(2*mass)) * density*(RPM^2)*pi*(R^4)*cos(pitch_cmd-flight_path), ...
    (-density/(2*mass)) * ( (airspeed^2)*Sref*CD_alpha + (RPM^2)*pi*(R^4)*throttle_cmd*sin(pitch_cmd-flight_path) ); ...
    (1/(2*airspeed)) * (density*(RPM^2)*pi*(R^4)*sin(pitch_cmd-flight_path)), ...
    (density/2) * (airspeed*Sref*CL_alpha + (1/airspeed)*(RPM^2)*pi*(R^4)*throttle_cmd*cos(pitch_cmd-flight_path) ) ];

== matlab function quadplane_control_dev/Subsystem1/LowPass Filter1/LP Filter on throttle outputs/MATLAB Function ==
  data: prev_val input single; raw_val input; filtered_val output; freq_cut input; samp_freq input
function filtered_val = IIR_filt( prev_val,raw_val, freq_cut, samp_freq)
    fc = freq_cut/samp_freq;
    b = 2 - cos(2 * pi * fc) - sqrt((2 - cos(2 * pi * fc))^2 - 1);
    a = 1 - b;
    filtered_val = a * raw_val + b * prev_val;

== matlab function quadplane_control_dev/FixedWing InnerLoop Control/INDI Based Angular Rate Controller/Calculate incremental term from INDI equation ==
  data: dynamic_pressure input; Sref input; bref input; cref input; Cl_coefs input; Cm_coefs input; Cn_coefs input; B_mat output single; inertia_matrix_inv input single
function B_mat = incremental_control_term(dynamic_pressure, Sref, bref, cref, Cl_coefs, Cm_coefs, Cn_coefs, inertia_matrix_inv)

% Format of the coefficients array is:: 
% [base_val, alpha, beta, p, q, r, aileron_def, elevator_def, rudder_def]

% deflections are [ail, elev, rudder]

% CY, Cl, Cn are functions of (beta, p, q, r, aileron_def, rudder_def)

% g(x) = inv(I) * moment contributions due to surface deflections
% this function calculates partial derivative of g wrt u (Jacobian). 

% just the jacobian with the coefficents and deflections
jacobian_g_wrt_u = [Cl_coefs(7), 0, Cl_coefs(9);...
    0, Cm_coefs(8), 0; ...
    Cn_coefs(7), 0, Cn_coefs(9)];

% including the total moments 
B_mat = inertia_matrix_inv * Sref * dynamic_pressure .* ...
    [bref, cref, bref]' .* jacobian_g_wrt_u;

== matlab function quadplane_control_dev/Hover Inner Loop/INDI inner loop/LowPass Filter1/LP Filter on throttle outputs/MATLAB Function ==
  data: prev_val input single; raw_val input; filtered_val output; freq_cut input; samp_freq input
function filtered_val = IIR_filt( prev_val,raw_val, freq_cut, samp_freq)
    fc = freq_cut/samp_freq;
    b = 2 - cos(2 * pi * fc) - sqrt((2 - cos(2 * pi * fc))^2 - 1);
    a = 1 - b;
    filtered_val = a * raw_val + b * prev_val;

== matlab function quadplane_control_dev/FixedWing OuterLoop Control/INDI Speed & Altitude Controller/MATLAB Function1 ==
  data: B0_mat input; x_ref_dot input; Kp_err_term input; del_u output; x_dot input
function del_u = incremental_output(B0_mat, x_ref_dot, Kp_err_term, x_dot)

% output equation of incremental INDI
del_u = B0_mat \ reshape((- x_dot + Kp_err_term + x_ref_dot), [2,1]);

== matlab function quadplane_control_dev/FixedWing InnerLoop Control/INDI Based Angular Rate Controller/LowPass Filter1/LP Filter on throttle outputs/MATLAB Function ==
  data: prev_val input single; raw_val input; filtered_val output; freq_cut input; samp_freq input
function filtered_val = IIR_filt( prev_val,raw_val, freq_cut, samp_freq)
    fc = freq_cut./samp_freq;
    b = 2 - cos(2 * pi .* fc) - sqrt((2 - cos(2 * pi .* fc)).^2 - 1);
    a = 1 - b;
    filtered_val = a .* raw_val + b .* prev_val;

== matlab function quadplane_control_dev/Hover Outer Loop/Speed Control/MATLAB Function ==
  data: roll_pitch input; B0_mat output; g input
function B0_mat = inversion_mat(roll_pitch, g)

roll = roll_pitch(1);
pitch = roll_pitch(2);

B0_mat = [0, -g*cos(pitch); g*cos(roll)*cos(pitch), -g*sin(roll)*sin(pitch)];

== matlab function quadplane_control_dev/Hover Outer Loop/Speed Control/MATLAB Function1 ==
  data: B0_mat input; y_ref_rate input; del_u output; error_term input; x_rate input
function del_u = indi_eqn(B0_mat, y_ref_rate, error_term, x_rate)

del_u = B0_mat \ (-x_rate + error_term + y_ref_rate);

== matlab function quadplane_control_dev/Hover Outer Loop/Altitude Control/MATLAB Function ==
  data: roll_pitch input; w_ref output; z_dot_nav_ref input
function w_ref = correct_att(roll_pitch, z_dot_nav_ref)

w_ref = z_dot_nav_ref / (cos(roll_pitch(1)) * cos(roll_pitch(2)));

== matlab function quadplane_control_dev/Check if speeding up/LowPass Filter/LP Filter on Accel/MATLAB Function ==
  data: prev_val input single; raw_val input; filtered_val output; freq_cut input; samp_freq input
function filtered_val = IIR_filt( prev_val,raw_val, freq_cut, samp_freq)
    fc = freq_cut ./ samp_freq;
    b = 2 - cos(2 * pi .* fc) - sqrt((2 - cos(2 * pi .* fc)).^2 - 1);
    a = 1 - b;
    filtered_val = a .* raw_val + b .* prev_val;

== matlab function quadplane_control_dev/Subsystem/motor_PWM_denormalize/remap ==
  data: norm_in input; raw_out output; in_min input; in_max input; out_min input; out_max input
function raw_out = remap(norm_in,in_min,in_max,out_min,out_max)
raw_out = (norm_in - in_min) * (out_max - out_min)/(in_max-in_min) + out_min;

== matlab function quadplane_control_dev/Hover Outer Loop/Conditioning/MATLAB Function ==
  data: u input; airspeed_cmd input; y output; speed_up_bool input; airspeed_cutoffs input
function y = reference_enabler(u, airspeed_cmd, speed_up_bool, airspeed_cutoffs)

y = single([0; 0]);
if speed_up_bool == 1 && airspeed_cmd <= airspeed_cutoffs(1)
    y = u; 
elseif speed_up_bool == 0 && airspeed_cmd <= airspeed_cutoffs(2)
    y = u;
else

end

== matlab function quadplane_control_dev/Hover Outer Loop/Speed Control/LowPass Filter2/LP Filter on throttle outputs/MATLAB Function ==
  data: prev_val input single; raw_val input; filtered_val output; freq_cut input; samp_freq input
function filtered_val = IIR_filt( prev_val,raw_val, freq_cut, samp_freq)
    fc = freq_cut/samp_freq;
    b = 2 - cos(2 * pi * fc) - sqrt((2 - cos(2 * pi * fc))^2 - 1);
    a = 1 - b;
    filtered_val = a * raw_val + b * prev_val;

== matlab function quadplane_control_dev/FixedWing OuterLoop Control/INDI Speed & Altitude Controller/LowPass Filter/LP Filter on Accel/MATLAB Function ==
  data: prev_val input single; raw_val input; filtered_val output; freq_cut input; samp_freq input
function filtered_val = IIR_filt( prev_val,raw_val, freq_cut, samp_freq)
    fc = freq_cut ./ samp_freq;
    b = 2 - cos(2 * pi .* fc) - sqrt((2 - cos(2 * pi .* fc)).^2 - 1);
    a = 1 - b;
    filtered_val = a .* raw_val + b .* prev_val;

== matlab function quadplane_control_dev/Mode Selection ==
  data: airspeed_cmd input; mode_input input; enable_hover output; enable_forward output; mode_changed output; mode output; sensors_active input; airspeed input; mode_shutoff_airspeeds input; prev_mode input
function [enable_hover, enable_forward, mode_changed, mode] = mode_selector(airspeed_cmd, mode_input, sensors_active, airspeed, mode_shutoff_airspeeds, prev_mode)

mode_changed = 0;

% event for mode input trigger (to figure out the transition type)
if prev_mode ~= mode_input
    mode_changed = 1;
end

if (sensors_active && mode_input==0)
    % Enable only Hover mode
    mode = 0;

elseif (sensors_active && mode_input==2)
    % Enable only forward flight mode
    mode = 2; 

% Need to be modified for real case use
elseif (sensors_active && mode_input==1)
    
    if airspeed_cmd < mode_shutoff_airspeeds(1) && airspeed < mode_shutoff_airspeeds(1) + 1
        mode = 0;
    elseif airspeed_cmd >= mode_shutoff_airspeeds(2) && airspeed >= mode_shutoff_airspeeds(2) + 1
        mode = 2;
    else
        mode = 1;
    end

elseif sensors_active && mode_input > 2
    error("Invalid mode selected ...")

else
    mode = 0;

end


% enable controllers for different modes
if mode == 0
    enable_hover = 1;
    enable_forward = 0;
elseif mode == 1
    enable_hover = 1;
    enable_forward = 1;
elseif mode == 2
    enable_hover = 0;
    enable_forward = 1;
else
    enable_hover = 0;
    enable_forward = 0;
end

== matlab function quadplane_control_dev/Enabled Subsystem/MATLAB Function ==
  data: alpha input; airspeed input; shutoff_airspeed input; adj_hover_thr output; adj_forward_thr output; hover_throttle input; forward_throttle input; surface_def input; adj_surface_def output; mode input
function [adj_hover_thr, adj_forward_thr, adj_surface_def] = weight_mixer(alpha, airspeed, shutoff_airspeed, hover_throttle, forward_throttle, surface_def, mode)

% adjusting the hover control outputs
adj_hover_thr = (1-alpha) .* hover_throttle;

% leaving the forward control outputs as is
adj_forward_thr = forward_throttle;
adj_surface_def = alpha .* surface_def;
% adj_surface_def = surface_def;

% disable inputs for diff modes. 
if mode == 0 
    adj_surface_def = single([0.0, 0.0, 0.0]');
    adj_forward_thr = single(0.0);
elseif mode == 2
    adj_hover_thr = single([0.0, 0.0, 0.0, 0.0]');
else
    % pass all control inputs
end

== matlab function quadplane_control_dev/Subsystem5/LowPass Filter1/LP Filter on throttle outputs/MATLAB Function ==
  data: prev_val input single; raw_val input; filtered_val output; freq_cut input; samp_freq input
function filtered_val = IIR_filt( prev_val,raw_val, freq_cut, samp_freq)
    fc = freq_cut/samp_freq;
    b = 2 - cos(2 * pi * fc) - sqrt((2 - cos(2 * pi * fc))^2 - 1);
    a = 1 - b;
    filtered_val = a * raw_val + b * prev_val;

== matlab function quadplane_control_dev/Subsystem/deflections_PWM_denormalize/remap ==
  data: norm_in input; raw_out output; in_min input; in_max input; out_min input; out_max input
function raw_out = remap(norm_in,in_min,in_max,out_min,out_max)
raw_out = (norm_in - in_min) * (out_max - out_min)/(in_max-in_min) + out_min;

== matlab function quadplane_control_dev/FixedWing InnerLoop Control/NDI based Attitude Controller/Changing euler angle rates to pqr ==
  data: yaw_rate_ref input; sum_term input; pqr_cmd output; roll_pitch input
function pqr_cmd = inversion_func(yaw_rate_ref, sum_term, roll_pitch)

roll = roll_pitch(1);
pitch = roll_pitch(2);

N_att_rates_to_pqr = [1, 0, -sin(pitch); ...
    0, cos(roll), sin(roll)*cos(pitch); ...
    0, -sin(roll), cos(roll)*cos(pitch)];

pqr_cmd = N_att_rates_to_pqr * [sum_term; yaw_rate_ref];

== matlab function quadplane_control_dev/FixedWing InnerLoop Control/INDI Based Angular Rate Controller/Calculate incremented input from INDI equation ==
  data: B_mat input; pqr_ref_dot input; del_u output; K_out input; pqr_dot input; yaw_damper input
function del_u = indi_input_calc(B_mat, pqr_ref_dot, K_out, pqr_dot, yaw_damper)

% INDI controller's change in output term
del_u = B_mat \ reshape((-pqr_dot + K_out + pqr_ref_dot), [3,1]);

% damping rudder output using the r-rate
del_u(3) = del_u(3) - yaw_damper * pqr_dot(3);
